simulink model "gm_Encoder_Zynq_V24"  (R2018a)
settings: Solver=ode3  StartTime=0.0  StopTime=SimulationsDauer  RelTol=1e-3  EnableMultiTasking=on
undefined symbols (not defined in the file or in its folder): DiscIntNeverNeededParam, f_ISR, IncPerTurn, n_max, OmegaPerOverSampl, OverSamplingFactor, OverSamplingFactorInverse, Periode, Phase_Delay_A, Phase_Delay_B, PolePair, QuadratureFactor, T_50MHz, T_mech, TestDrehzahl_rpm
libraries: simulink x2, dspswit3 x2, powerlib_meascontrol x2, simulink_extras x1, powerlib x1
(part 3 of 4)

== system gm_Encoder_Zynq_V24/IncreEncoder_V22/omega_by_measure_time ==
  note: Use new Speed after every positive A-Line Edge
  note: 1 for one cycle if edge recognized
  note: Detect each positive edge of the A-Line of the encoder
  note: Reset time measurement
  note: Count up in order to measure the time between to positive edges of the A-Line of the encoder
  Edge : Inport
  T : Inport  Port=2
  Add1 : Sum  OutDataTypeStr=Inherit: Same as first input
  Constant : Constant  Value=0  OutDataTypeStr=fixdt(0,32,26)  SampleTime=-1
  Constant1 : Constant  Value=0  OutDataTypeStr=fixdt(0,32,26)  SampleTime=-1
  Constant2 : Constant  Value=0  OutDataTypeStr=fixdt(0,32,26)  SampleTime=-1
  Constant3 : Constant  Value=0  OutDataTypeStr=int8  SampleTime=-1
  Detec_edge : Sum  Inputs=+-  AccumDataTypeStr=int8  OutDataTypeStr=int8
  ProtectOverflow_T_count : Switch  Threshold=50
  ProtectOverflow_rps : Switch  Threshold=50  OutDataTypeStr=fixdt(0,32,26)
  ProtectToUseOmegaIfThetaJump1 : RelationalOperator  Operator=>  OutDataTypeStr=boolean  RndMeth=Nearest
  Scope : Scope  NumInputPorts=3
  T_count : Delay  DelayLength=1
  T_count_switch : Switch  Criteria=u2 > Threshold
  count_old1 : Delay  DelayLength=1
  reset_old1 : Delay  DelayLength=1
  reset_old_switch1 : Switch  Criteria=u2 ~= 0
  speed_old : Delay  DelayLength=1
  speed_old_switch : Switch  Criteria=u2 ~= 0  OutDataTypeStr=fixdt(0,32,26)  RndMeth=Zero
  rps : Outport
  NewMeasurement : Outport  Port=2
  wires:
  Detec_edge/1 -> reset_old_switch1/2, count_old1/1  "1 for one cycle if edge recognized"
  reset_old1/1 -> Detec_edge/2, reset_old_switch1/3
  reset_old_switch1/1 -> reset_old1/1
  Edge/1 -> Detec_edge/1, reset_old_switch1/1
  ProtectToUseOmegaIfThetaJump1/1 -> T_count_switch/2, speed_old_switch/2, NewMeasurement/1, Scope/1
  Constant3/1 -> ProtectToUseOmegaIfThetaJump1/2
  count_old1/1 -> ProtectToUseOmegaIfThetaJump1/1
  T_count_switch/1 -> ProtectOverflow_T_count/2, ProtectOverflow_T_count/3, ProtectOverflow_rps/2
  Add1/1 -> T_count_switch/3, speed_old_switch/1, Scope/2
  T_count/1 -> Add1/2
  ProtectOverflow_T_count/1 -> T_count/1
  T/1 -> Add1/1
  speed_old/1 -> speed_old_switch/3
  speed_old_switch/1 -> speed_old/1, ProtectOverflow_rps/3
  Constant2/1 -> ProtectOverflow_rps/1
  ProtectOverflow_rps/1 -> rps/1, Scope/3
  Constant1/1 -> ProtectOverflow_T_count/1
  Constant/1 -> T_count_switch/1

== system gm_Encoder_Zynq_V24/IncreEncoder_V24/Check_Direction ==
  A : Inport  PortDimensions=1  SampleTime=2e-08
  B : Inport  Port=2  PortDimensions=1  SampleTime=2e-08
  Add : Sum  Inputs=+-  AccumDataTypeStr=fixdt(1, 4, 0)  OutDataTypeStr=fixdt(1, 4, 0)  SampleTime=2e-08
  Add1 : Sum  Inputs=+-  AccumDataTypeStr=fixdt(1, 4, 0)  OutDataTypeStr=fixdt(1, 4, 0)  SampleTime=2e-08
  Add2 : Sum  AccumDataTypeStr=fixdt(1, 4, 0)  OutDataTypeStr=fixdt(1, 4, 0)  SampleTime=2e-08
  Change : Sum  AccumDataTypeStr=fixdt(1, 4, 0)  OutDataTypeStr=fixdt(1, 4, 0)  SampleTime=2e-08
  Change1 : Delay  DelayLength=double(1)  InitialCondition=0  InputProcessing=Inherited  SampleTime=2e-08
  Save_Direction : Switch  Criteria=u2 ~= 0  Threshold=double(0)  OutDataTypeStr=fixdt(1, 4, 0)  SampleTime=2e-08
  T_count_switch : Switch  Threshold=double(1)  OutDataTypeStr=fixdt(1, 4, 0)  SampleTime=2e-08
  TrnLeft : Sum  Inputs=+-  AccumDataTypeStr=fixdt(1, 4, 0)  OutDataTypeStr=fixdt(1, 4, 0)  SampleTime=2e-08
  TrnRight : Sum  Inputs=+-  AccumDataTypeStr=fixdt(1, 4, 0)  OutDataTypeStr=fixdt(1, 4, 0)  SampleTime=2e-08
  TurnLeft : Constant  Value=fi(0,1,4,0,'hex','f')  OutDataTypeStr=fixdt(1, 4, 0)  SampleTime=-1
  TurnRight : Constant  Value=fi(0,1,4,0,'hex','1')  OutDataTypeStr=fixdt(1, 4, 0)  SampleTime=-1
  count_old : Delay  DelayLength=double(1)  InitialCondition=0  InputProcessing=Inherited  SampleTime=2e-08
  count_old1 : Delay  DelayLength=double(1)  InitialCondition=0  InputProcessing=Inherited  SampleTime=2e-08
  count_old2 : Delay  DelayLength=double(1)  InitialCondition=0  InputProcessing=Inherited  SampleTime=2e-08
  count_old_switch : Switch  Criteria=u2 ~= 0  Threshold=double(0)  OutDataTypeStr=boolean  SampleTime=2e-08
  count_old_switch1 : Switch  Criteria=u2 ~= 0  Threshold=double(0)  OutDataTypeStr=boolean  SampleTime=2e-08
  new_value : Delay  DelayLength=double(1)  InitialCondition=0  InputProcessing=Inherited  SampleTime=2e-08
  nothing : Constant  Value=fi(0,1,4,0,'hex','0')  OutDataTypeStr=fixdt(1, 4, 0)  SampleTime=-1
  nothing1 : Constant  Value=fi(0,1,4,0,'hex','0')  OutDataTypeStr=fixdt(1, 4, 0)  SampleTime=-1
  speed_old_switch : Switch  Threshold=double(1)  OutDataTypeStr=fixdt(1, 4, 0)  SampleTime=2e-08
  Dir : Outport
  wires:
  A/1 -> TrnLeft/2, Add/1, count_old_switch/1
  B/1 -> TrnRight/2, Add1/1, count_old_switch1/1
  Add/1 -> TrnRight/1, count_old_switch/2
  Add1/1 -> TrnLeft/1, count_old_switch1/2
  Add2/1 -> new_value/1
  Change/1 -> Change1/1
  Change1/1 -> Save_Direction/2
  T_count_switch/1 -> Change/1, Add2/1
  TrnLeft/1 -> speed_old_switch/2
  TrnRight/1 -> T_count_switch/2
  TurnLeft/1 -> speed_old_switch/1
  TurnRight/1 -> T_count_switch/1
  count_old2/1 -> Dir/1, Save_Direction/3
  new_value/1 -> Save_Direction/1
  nothing/1 -> speed_old_switch/3
  nothing1/1 -> T_count_switch/3
  speed_old_switch/1 -> Change/2, Add2/2
  count_old_switch/1 -> count_old/1
  count_old/1 -> count_old_switch/3, Add/2
  count_old_switch1/1 -> count_old1/1
  count_old1/1 -> count_old_switch1/3, Add1/2
  Save_Direction/1 -> count_old2/1

== system gm_Encoder_Zynq_V24/IncreEncoder_V24/Counter ==
  note: Reset
  note: 1 for one cycle if edge recognized
  Enable_ctr : Inport  PortDimensions=1  SampleTime=2e-08
  I_line : Inport  Port=2  PortDimensions=1  SampleTime=2e-08
  Detec_edge : Sum  Inputs=+-  AccumDataTypeStr=int8  OutDataTypeStr=int8  SampleTime=2e-08
  Reset_flag : Sum  Inputs=+-  AccumDataTypeStr=uint8  OutDataTypeStr=uint8  SampleTime=2e-08
  reset_old : Delay  DelayLength=double(1)  InitialCondition=0  InputProcessing=Inherited  SampleTime=2e-08
  reset_old1 : Delay  DelayLength=double(1)  InitialCondition=0  InputProcessing=Inherited  SampleTime=2e-08
  reset_old_switch : Switch  Criteria=u2 ~= 0  Threshold=double(0)  OutDataTypeStr=boolean  SampleTime=2e-08
  reset_old_switch1 : Switch  Criteria=u2 ~= 0  Threshold=double(0)  OutDataTypeStr=boolean  SampleTime=2e-08
  Edge : Outport
  Reset : Outport  Port=2
  wires:
  Enable_ctr/1 -> Detec_edge/1, reset_old_switch1/1
  I_line/1 -> Reset_flag/1, reset_old_switch/1
  Detec_edge/1 -> Edge/1, reset_old_switch1/2
  Reset_flag/1 -> Reset/1, reset_old_switch/2
  reset_old_switch1/1 -> reset_old1/1
  reset_old1/1 -> reset_old_switch1/3, Detec_edge/2
  reset_old_switch/1 -> reset_old/1
  reset_old/1 -> reset_old_switch/3, Reset_flag/2

== system gm_Encoder_Zynq_V24/IncreEncoder_V24/Counter_position ==
  note: Check if count is to small
  note: Check if count is to big 0-Increments
  note: Count
  Edge : Inport  PortDimensions=1  SampleTime=2e-08
  Reset : Inport  Port=2  PortDimensions=1  SampleTime=2e-08
  IncsPerTurn : Inport  Port=3  PortDimensions=1  SampleTime=2e-08
  Dir : Inport  Port=4  PortDimensions=1  SampleTime=2e-08
  Add1 : Sum  AccumDataTypeStr=int16  OutDataTypeStr=int16  SampleTime=2e-08
  Constant1 : Constant  Value=fi(0,1,16,0,'hex','0000')  OutDataTypeStr=int16  SampleTime=-1
  Constant2 : Constant  Value=fi(0,1,16,0,'hex','0001')  OutDataTypeStr=int16  SampleTime=-1
  Constant3 : Constant  Value=fi(0,1,16,0,'hex','0000')  OutDataTypeStr=int16  SampleTime=-1
  Constant5 : Constant  Value=fi(0,1,16,0,'hex','ffff')  OutDataTypeStr=int16  SampleTime=-1
  Relational Operator : RelationalOperator  Operator=>  OutDataTypeStr=boolean  SampleTime=2e-08  RndMeth=Nearest
  Relational Operator1 : RelationalOperator  Operator=<=  OutDataTypeStr=boolean  SampleTime=2e-08  RndMeth=Nearest
  Resett_switch1 : Switch  Criteria=u2 ~= 0  Threshold=double(0)  OutDataTypeStr=uint16  SampleTime=2e-08
  Resett_switch2 : Switch  Criteria=u2 ~= 0  Threshold=double(0)  OutDataTypeStr=int16  SampleTime=2e-08
  Resett_switch3 : Switch  Criteria=u2 ~= 0  Threshold=double(0)  OutDataTypeStr=int16  SampleTime=2e-08
  only_use_for_neg_speed : Switch  Threshold=double(1)  OutDataTypeStr=int16  SampleTime=2e-08
  reset_old{1..6} (6 alike) : Delay  DelayLength=double(1)  InitialCondition=0  InputProcessing=Inherited  SampleTime=2e-08
  speed_old_switch1 : Switch  Criteria=u2 ~= 0  Threshold=double(0)  OutDataTypeStr=int16  SampleTime=2e-08
  speed_old_switch2 : Switch  Threshold=double(1)  OutDataTypeStr=int16  SampleTime=2e-08
  count : Outport
  wires:
  Edge/1 -> speed_old_switch1/2
  Reset/1 -> Resett_switch2/2
  IncsPerTurn/1 -> reset_old5/1
  Dir/1 -> reset_old6/1
  Constant1/1 -> Relational Operator1/2, Resett_switch1/1, Resett_switch2/1, only_use_for_neg_speed/1
  Constant2/1 -> speed_old_switch2/1
  Constant3/1 -> speed_old_switch1/3
  Constant5/1 -> speed_old_switch2/3
  Resett_switch1/1 -> count/1, reset_old1/1, Relational Operator/1
  reset_old4/1 -> speed_old_switch1/1
  reset_old5/1 -> Relational Operator/2, Resett_switch3/1
  reset_old6/1 -> speed_old_switch2/2, only_use_for_neg_speed/2
  speed_old_switch1/1 -> Add1/1
  speed_old_switch2/1 -> reset_old4/1
  Resett_switch2/1 -> Resett_switch3/3
  Add1/1 -> Resett_switch2/3
  reset_old1/1 -> Add1/2
  Relational Operator1/1 -> reset_old2/1
  reset_old2/1 -> only_use_for_neg_speed/3
  only_use_for_neg_speed/1 -> Resett_switch3/2
  Resett_switch3/1 -> Resett_switch1/3, Relational Operator1/1
  Relational Operator/1 -> reset_old3/1
  reset_old3/1 -> Resett_switch1/2

== system gm_Encoder_Zynq_V24/IncreEncoder_V24/Counter_theta_ele ==
  note: Check if count is to small
  note: Count
  Edge : Inport  PortDimensions=1  SampleTime=2e-08
  Reset : Inport  Port=2  PortDimensions=1  SampleTime=2e-08
  IncsPerTurn : Inport  Port=3  PortDimensions=1  SampleTime=2e-08
  Dir : Inport  Port=4  PortDimensions=1  SampleTime=2e-08
  Add1 : Sum  AccumDataTypeStr=int16  OutDataTypeStr=int16  SampleTime=2e-08
  Constant1 : Constant  Value=fi(0,1,16,0,'hex','0000')  OutDataTypeStr=int16  SampleTime=-1
  Constant2 : Constant  Value=fi(0,1,16,0,'hex','0001')  OutDataTypeStr=int16  SampleTime=-1
  Constant3 : Constant  Value=fi(0,1,16,0,'hex','0000')  OutDataTypeStr=int16  SampleTime=-1
  Constant5 : Constant  Value=fi(0,1,16,0,'hex','ffff')  OutDataTypeStr=int16  SampleTime=-1
  Relational Operator : RelationalOperator  Operator=>  OutDataTypeStr=boolean  SampleTime=2e-08  RndMeth=Nearest
  Relational Operator1 : RelationalOperator  Operator=<=  OutDataTypeStr=boolean  SampleTime=2e-08  RndMeth=Nearest
  Reset_switch3 : Switch  Criteria=u2 ~= 0  Threshold=double(0)  OutDataTypeStr=int16  SampleTime=2e-08
  Resett_switch1 : Switch  Criteria=u2 ~= 0  Threshold=double(0)  OutDataTypeStr=int16  SampleTime=2e-08
  Resett_switch2 : Switch  Criteria=u2 ~= 0  Threshold=double(0)  OutDataTypeStr=int16  SampleTime=2e-08
  only_use_for_neg_speed : Switch  Threshold=double(1)  OutDataTypeStr=int16  SampleTime=2e-08
  reset_old{1..6} (6 alike) : Delay  DelayLength=double(1)  InitialCondition=0  InputProcessing=Inherited  SampleTime=2e-08
  speed_old_switch1 : Switch  Criteria=u2 ~= 0  Threshold=double(0)  OutDataTypeStr=int16  SampleTime=2e-08
  speed_old_switch2 : Switch  Threshold=double(1)  OutDataTypeStr=int16  SampleTime=2e-08
  count : Outport
  wires:
  Edge/1 -> speed_old_switch1/2
  Reset/1 -> Resett_switch2/2
  IncsPerTurn/1 -> reset_old1/1
  Dir/1 -> reset_old5/1
  Constant1/1 -> Relational Operator1/2, Resett_switch1/1, Resett_switch2/1, only_use_for_neg_speed/1
  Constant2/1 -> speed_old_switch2/1
  Constant3/1 -> speed_old_switch1/3
  Constant5/1 -> speed_old_switch2/3
  Resett_switch1/1 -> count/1, reset_old6/1, Relational Operator/1
  reset_old1/1 -> Relational Operator/2, Reset_switch3/1
  reset_old4/1 -> speed_old_switch1/1
  reset_old5/1 -> speed_old_switch2/2, only_use_for_neg_speed/2
  speed_old_switch1/1 -> Add1/1
  speed_old_switch2/1 -> reset_old4/1
  Resett_switch2/1 -> Reset_switch3/3
  Add1/1 -> Resett_switch2/3
  reset_old6/1 -> Add1/2
  Relational Operator1/1 -> reset_old2/1
  reset_old2/1 -> only_use_for_neg_speed/3
  only_use_for_neg_speed/1 -> Reset_switch3/2
  Reset_switch3/1 -> Resett_switch1/3, Relational Operator1/1
  Relational Operator/1 -> reset_old3/1
  reset_old3/1 -> Resett_switch1/2

== system gm_Encoder_Zynq_V24/IncreEncoder_V24/HDL Reciprocal ==
  In1 : Inport
  Delay1 : Delay  DelayLength=1  InputProcessing=Inherited
  Delay2 : Delay  DelayLength=3  InputProcessing=Inherited
  HDL Reciprocal : Reciprocal  SampleTime=2e-08
  Out1 : Outport
  wires:
  In1/1 -> Delay1/1
  Delay1/1 -> HDL Reciprocal/1
  HDL Reciprocal/1 -> Delay2/1
  Delay2/1 -> Out1/1

== system gm_Encoder_Zynq_V24/IncreEncoder_V24/omega_by_count_lines ==
  note: Count
  note: Check if count is to big in order to safe for value overflow
  note: Set new counter value
  Edge : Inport  PortDimensions=1  SampleTime=2e-08
  Reset : Inport  Port=2  PortDimensions=1  SampleTime=2e-08
  IncsPerTurn : Inport  Port=3  PortDimensions=1  SampleTime=2e-08
  Add1 : Sum  AccumDataTypeStr=int16  OutDataTypeStr=int16  SampleTime=2e-08
  Constant1 : Constant  Value=fi(0,1,16,0,'hex','0000')  OutDataTypeStr=int16  SampleTime=-1
  Constant2 : Constant  Value=fi(0,1,16,0,'hex','0001')  OutDataTypeStr=int16  SampleTime=-1
  Constant3 : Constant  Value=fi(0,1,16,0,'hex','0000')  OutDataTypeStr=int16  SampleTime=-1
  Constant4 : Constant  Value=fi(0,1,16,0,'hex','000a')  OutDataTypeStr=int16  SampleTime=-1
  Relational Operator : RelationalOperator  Operator=>  OutDataTypeStr=boolean  SampleTime=2e-08  RndMeth=Nearest
  Reset_when_overflow : Sum  AccumDataTypeStr=fixdt(1, 18, 0)  OutDataTypeStr=int16  SampleTime=2e-08
  Resett_switch1 : Switch  Criteria=u2 ~= 0  Threshold=double(0)  OutDataTypeStr=int16  SampleTime=2e-08
  Resett_switch2 : Switch  Criteria=u2 ~= 0  Threshold=double(0)  OutDataTypeStr=int16  SampleTime=2e-08
  reset_old{1,3..5} (4 alike) : Delay  DelayLength=double(1)  InitialCondition=0  InputProcessing=Inherited  SampleTime=2e-08
  reset_old_switch1 : Switch  Criteria=u2 ~= 0  Threshold=double(0)  OutDataTypeStr=int16  SampleTime=2e-08
  speed_old_switch1 : Switch  Criteria=u2 ~= 0  Threshold=double(0)  OutDataTypeStr=int16  SampleTime=2e-08
  count : Outport
  wires:
  Edge/1 -> speed_old_switch1/2
  Reset/1 -> Resett_switch2/2, reset_old_switch1/2
  IncsPerTurn/1 -> Reset_when_overflow/2
  Constant1/1 -> Resett_switch1/1, Resett_switch2/1
  Constant2/1 -> reset_old4/1
  Constant3/1 -> speed_old_switch1/3
  Constant4/1 -> Reset_when_overflow/1
  Reset_when_overflow/1 -> reset_old5/1
  reset_old3/1 -> Add1/2, Relational Operator/1, reset_old_switch1/1
  reset_old4/1 -> speed_old_switch1/1
  reset_old5/1 -> Relational Operator/2
  reset_old_switch1/1 -> count/1, reset_old1/1
  speed_old_switch1/1 -> Add1/1
  Resett_switch2/1 -> Resett_switch1/3
  Add1/1 -> Resett_switch2/3
  Relational Operator/1 -> Resett_switch1/2
  Resett_switch1/1 -> reset_old3/1
  reset_old1/1 -> reset_old_switch1/3

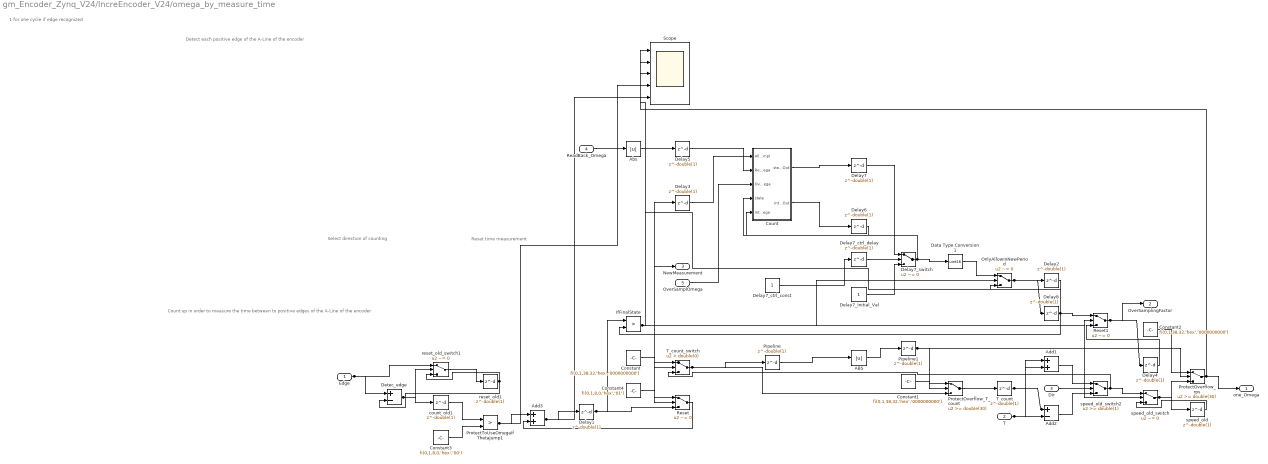
== system gm_Encoder_Zynq_V24/IncreEncoder_V24/omega_by_measure_time ==
  note: Select direction of counting
  note: 1 for one cycle if edge recognized
  note: Detect each positive edge of the A-Line of the encoder
  note: Reset time measurement
  note: Count up in order to measure the time between to positive edges of the A-Line of the encoder
  Edge : Inport  PortDimensions=1  SampleTime=2e-08
  T : Inport  Port=2  PortDimensions=1  SampleTime=2e-08
  Dir : Inport  Port=3  PortDimensions=1  SampleTime=2e-08
  ReadBack_Omega : Inport  Port=4  PortDimensions=1  SampleTime=2e-08
  OverSamplOmega : Inport  Port=5  PortDimensions=1  SampleTime=2e-08
  ABS : Abs  SampleTime=2e-08  OutDataTypeStr=fixdt(1, 38, 32)
  Abs : Abs  SampleTime=2e-08  OutDataTypeStr=fixdt(1, 24, 11)
  Add1 : Sum  AccumDataTypeStr=fixdt(1, 38, 32)  OutDataTypeStr=fixdt(1, 38, 32)  SampleTime=2e-08
  Add2 : Sum  Inputs=+-  AccumDataTypeStr=fixdt(1, 38, 32)  OutDataTypeStr=fixdt(1, 38, 32)  SampleTime=2e-08
  Add3 : Sum  AccumDataTypeStr=int16  OutDataTypeStr=int16  SampleTime=2e-08
  Constant : Constant  Value=fi(0,1,38,32,'hex','0000000000')  OutDataTypeStr=fixdt(1, 38, 32)  SampleTime=-1
  Constant1 : Constant  Value=fi(0,1,38,32,'hex','0000000000')  OutDataTypeStr=fixdt(1, 38, 32)  SampleTime=-1
  Constant2 : Constant  Value=fi(0,1,38,32,'hex','0000000000')  OutDataTypeStr=fixdt(1, 38, 32)  SampleTime=-1
  Constant3 : Constant  Value=fi(0,1,8,0,'hex','00')  OutDataTypeStr=int8  SampleTime=-1
  Constant4 : Constant  Value=fi(0,1,8,0,'hex','01')  OutDataTypeStr=int8  SampleTime=-1
  Count : Subsystem
  Data Type Conversion1 : DataTypeConversion  OutDataTypeStr=uint16  SampleTime=2e-08
  Delay{1..8} (8 alike) : Delay  DelayLength=double(1)  InitialCondition=0  InputProcessing=Inherited  SampleTime=2e-08
  Delay7_Initial_Val : Constant  OutDataTypeStr=uint16  SampleTime=-1
  Delay7_ctrl_const : Constant  OutDataTypeStr=boolean  SampleTime=2e-08
  Delay7_ctrl_delay : Delay  DelayLength=double(1)  InitialCondition=0  InputProcessing=Inherited  SampleTime=2e-08
  Delay7_switch : Switch  Criteria=u2 ~= 0  Threshold=double(0)  OutDataTypeStr=uint16  SampleTime=2e-08
  Detec_edge : Sum  Inputs=+-  AccumDataTypeStr=int8  OutDataTypeStr=int8  SampleTime=2e-08
  IfFinalState : RelationalOperator  Operator=>  OutDataTypeStr=boolean  SampleTime=2e-08  RndMeth=Nearest
  OnlyAllowInNewPeriod : Switch  Criteria=u2 ~= 0  Threshold=double(0)  OutDataTypeStr=uint16  SampleTime=2e-08
  Pipeline : Delay  DelayLength=double(1)  InitialCondition=0  InputProcessing=Inherited  SampleTime=2e-08
  Pipeline1 : Delay  DelayLength=double(1)  InitialCondition=0  InputProcessing=Inherited  SampleTime=2e-08
  ProtectOverflow_T_count : Switch  Threshold=double(30)  OutDataTypeStr=fixdt(1, 38, 32)  SampleTime=2e-08
  ProtectOverflow_rps : Switch  Threshold=double(30)  OutDataTypeStr=fixdt(1, 38, 32)  SampleTime=2e-08
  ProtectToUseOmegaIfThetaJump1 : RelationalOperator  Operator=>  SampleTime=2e-08  RndMeth=Nearest
  Reset : Switch  Criteria=u2 ~= 0  Threshold=double(0)  OutDataTypeStr=fixdt(1, 24, 11)  SampleTime=2e-08
  Reset1 : Switch  Criteria=u2 ~= 0  Threshold=double(0)  OutDataTypeStr=uint16  SampleTime=2e-08
  Scope : Scope  NumInputPorts=5
  T_count : Delay  DelayLength=double(1)  InitialCondition=0  InputProcessing=Inherited  SampleTime=2e-08
  T_count_switch : Switch  Criteria=u2 > Threshold  Threshold=double(0)  OutDataTypeStr=fixdt(1, 38, 32)  SampleTime=2e-08
  count_old1 : Delay  DelayLength=double(1)  InitialCondition=0  InputProcessing=Inherited  SampleTime=2e-08
  reset_old1 : Delay  DelayLength=double(1)  InitialCondition=0  InputProcessing=Inherited  SampleTime=2e-08
  reset_old_switch1 : Switch  Criteria=u2 ~= 0  Threshold=double(0)  OutDataTypeStr=boolean  SampleTime=2e-08
  speed_old : Delay  DelayLength=double(1)  InitialCondition=0  InputProcessing=Inherited  SampleTime=2e-08
  speed_old_switch : Switch  Criteria=u2 ~= 0  Threshold=double(0)  OutDataTypeStr=fixdt(1, 38, 32)  SampleTime=2e-08
  speed_old_switch2 : Switch  Threshold=double(1)  OutDataTypeStr=fixdt(1, 38, 32)  SampleTime=2e-08
  one_Omega : Outport
  OverSamplingFactor : Outport  Port=2
  NewMeasurement : Outport  Port=3
  wires:
  Edge/1 -> reset_old_switch1/1, Detec_edge/1
  T/1 -> Add2/2, Add1/2
  Dir/1 -> speed_old_switch2/2
  ReadBack_Omega/1 -> Abs/1
  OverSamplOmega/1 -> Count/3(OverSamplOmega)
  ABS/1 -> Pipeline1/1
  Abs/1 -> Delay5/1
  Add1/1 -> speed_old_switch2/1
  Add2/1 -> speed_old_switch2/3
  Add3/1 -> Scope/5, Delay1/1
  Constant/1 -> T_count_switch/1
  Constant1/1 -> ProtectOverflow_T_count/1
  Constant2/1 -> ProtectOverflow_rps/1
  Constant3/1 -> ProtectToUseOmegaIfThetaJump1/2
  Constant4/1 -> Reset/1
  Count/1(state_Out) -> Delay7/1
  Count/2(InternalOmega_Out) -> Delay6/1
  Data Type Conversion1/1 -> OnlyAllowInNewPeriod/1
  Delay1/1 -> Reset/3, IfFinalState/1
  Delay2/1 -> OnlyAllowInNewPeriod/3
  Delay3/1 -> Count/1(AllowCheckOverSampl)
  Delay4/1 -> Reset1/3
  Delay5/1 -> Count/2(ReadBack_Omega)
  Delay6/1 -> Count/5(InternalOmega)
  Delay7_switch/1 -> Data Type Conversion1/1, Count/4(state)
  Delay8/1 -> Reset1/1, IfFinalState/2, Scope/2
  Detec_edge/1 -> reset_old_switch1/2, count_old1/1
  IfFinalState/1 -> speed_old_switch/2, T_count_switch/2, Reset1/2, Reset/2, OnlyAllowInNewPeriod/2, Scope/1, Delay3/1, NewMeasurement/1
  OnlyAllowInNewPeriod/1 -> Delay8/1, Delay2/1
  Pipeline/1 -> ABS/1
  Pipeline1/1 -> ProtectOverflow_rps/2, ProtectOverflow_T_count/2
  ProtectOverflow_T_count/1 -> T_count/1
  ProtectOverflow_rps/1 -> Scope/3, one_Omega/1
  ProtectToUseOmegaIfThetaJump1/1 -> Add3/1, Scope/4
  Reset/1 -> Add3/2
  Reset1/1 -> Delay4/1, OverSamplingFactor/1
  T_count/1 -> Add2/1, Add1/1
  T_count_switch/1 -> ProtectOverflow_T_count/3, Pipeline/1
  count_old1/1 -> ProtectToUseOmegaIfThetaJump1/1
  reset_old1/1 -> reset_old_switch1/3, Detec_edge/2
  reset_old_switch1/1 -> reset_old1/1
  speed_old/1 -> speed_old_switch/3
  speed_old_switch/1 -> ProtectOverflow_rps/3, speed_old/1
  speed_old_switch2/1 -> speed_old_switch/1, T_count_switch/3
  Delay7/1 -> Delay7_switch/1
  Delay7_Initial_Val/1 -> Delay7_switch/3
  Delay7_ctrl_const/1 -> Delay7_ctrl_delay/1
  Delay7_ctrl_delay/1 -> Delay7_switch/2

== system gm_Encoder_Zynq_V24/IncreEncoder_V24_Gut/Average ==
  note: Maximum of the OverSampling is 6
  "OmegaIn " : Inport
  NewMeasurement : Inport  Port=2
  SamplingFactorInv : Inport  Port=3
  SamplingFactor : Inport  Port=4
  Add : Sum  Inputs=++++++  AccumDataTypeStr=fixdt(1,26,11)  OutDataTypeStr=fixdt(1,25,11)
  Ask1 : Switch  Threshold=fi(2,0,4,0)  OutDataTypeStr=fixdt(1,24,11)
  Ask2 : Switch  Threshold=fi(3,0,4,0)  OutDataTypeStr=fixdt(1,24,11)
  Ask3 : Switch  Threshold=fi(4,0,4,0)  OutDataTypeStr=fixdt(1,24,11)
  Ask4 : Switch  Threshold=fi(5,0,4,0)  OutDataTypeStr=fixdt(1,24,11)
  Ask5 : Switch  Threshold=fi(6,0,4,0)  OutDataTypeStr=fixdt(1,24,11)
  Constant1 : Constant  Value=0  OutDataTypeStr=fixdt(1,24,11)  SampleTime=-1
  NewSpeed{,1..4} (5 alike) : Switch  Criteria=u2 ~= 0  Threshold=0.5  OutDataTypeStr=fixdt(1,24,11)
  Product : Product  OutDataTypeStr=fixdt(1,24,11)
  hold{,1..4} (5 alike) : Delay  DelayLength=1
  OmegaOut : Outport
  wires:
  SamplingFactor/1 -> Ask5/2, Ask4/2, Ask3/2, Ask2/2, Ask1/2
  Ask5/1 -> Add/6
  Ask4/1 -> Add/5
  Ask3/1 -> Add/4
  Ask2/1 -> Add/3
  Ask1/1 -> Add/2
  Constant1/1 -> Ask1/3, Ask2/3, Ask3/3, Ask4/3, Ask5/3
  hold4/1 -> NewSpeed4/3
  NewSpeed4/1 -> Ask5/1, hold4/1
  hold3/1 -> NewSpeed3/3, NewSpeed4/1
  NewSpeed3/1 -> Ask4/1, hold3/1
  NewMeasurement/1 -> NewSpeed1/2, NewSpeed2/2, NewSpeed3/2, NewSpeed4/2, NewSpeed/2
  NewSpeed2/1 -> Ask3/1, hold2/1
  hold2/1 -> NewSpeed2/3, NewSpeed3/1
  hold1/1 -> NewSpeed1/3, NewSpeed2/1
  NewSpeed1/1 -> Ask2/1, hold1/1
  NewSpeed/1 -> Ask1/1, hold/1
  hold/1 -> NewSpeed/3, NewSpeed1/1
  Add/1 -> Product/1
  SamplingFactorInv/1 -> Product/2
  "OmegaIn "/1 -> NewSpeed/1, Add/1
  Product/1 -> OmegaOut/1

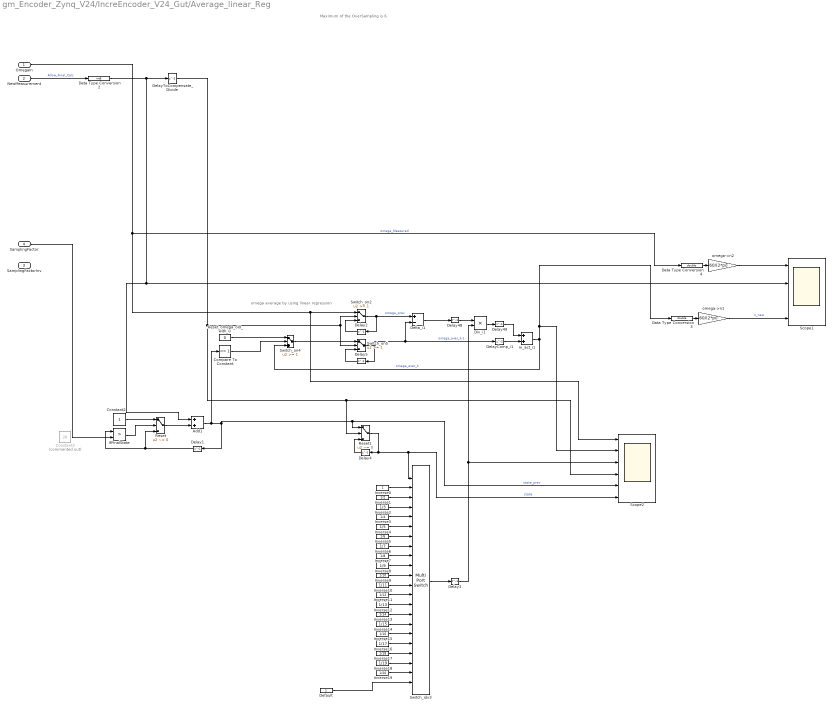
== system gm_Encoder_Zynq_V24/IncreEncoder_V24_Gut/Average_linear_Reg ==
  note: omega average by using linear regression
  note: Maximum of the OverSampling is 6
  "OmegaIn " : Inport
  NewMeasurement : Inport  Port=2
  SamplingFactorInv : Inport  Port=3
  SamplingFactor : Inport  Port=4
  Add1 : Sum  OutDataTypeStr=Inherit: Same as accumulator
  Compare To Constant : simulink/Logic and Bit Operations/Compare To Constant  relop===  const=1  OutDataTypeStr=boolean
  Constant2 : Constant  OutDataTypeStr=int8  SampleTime=T_50MHz
  Constant3 : Constant  Commented=on  Value=20  OutDataTypeStr=uint16  SampleTime=T_50MHz
  Data Type Conversion2 : DataTypeConversion  OutDataTypeStr=int8
  Data Type Conversion3 : DataTypeConversion  OutDataTypeStr=double
  Data Type Conversion4 : DataTypeConversion  OutDataTypeStr=double
  Default : Constant  OutDataTypeStr=fixdt(0,18,18)  SampleTime=-1
  Delay{1..5,48..49} (7 alike) : Delay  DelayLength=1  InitialCondition=0
  DelayComp_i1 : Delay  InitialCondition=0
  DelayToCompensate_Divide : Delay
  Delta_i1 : Sum  Inputs=+-  AccumDataTypeStr=fixdt(1,32,18)  OutDataTypeStr=fixdt(1,24,11)
  Div_i1 : Product  Inputs=**  RndMeth=Simplest  SaturateOnIntegerOverflow=on  OutDataTypeStr=Inherit: Same as first input
  IfFinalState : RelationalOperator  Operator=>  OutDataTypeStr=boolean  RndMeth=Nearest
  Inverse0 : Constant  OutDataTypeStr=fixdt(0,18,18)  SampleTime=-1
  Inverse1 : Constant  Value=1/2  OutDataTypeStr=fixdt(0,18,18)  SampleTime=-1
  Inverse10 : Constant  Value=1/11  OutDataTypeStr=fixdt(0,18,18)  SampleTime=-1
  Inverse11 : Constant  Value=1/12  OutDataTypeStr=fixdt(0,18,18)  SampleTime=-1
  Inverse12 : Constant  Value=1/13  OutDataTypeStr=fixdt(0,18,18)  SampleTime=-1
  Inverse13 : Constant  Value=1/14  OutDataTypeStr=fixdt(0,18,18)  SampleTime=-1
  Inverse14 : Constant  Value=1/15  OutDataTypeStr=fixdt(0,18,18)  SampleTime=-1
  Inverse15 : Constant  Value=1/16  OutDataTypeStr=fixdt(0,18,18)  SampleTime=-1
  Inverse16 : Constant  Value=1/17  OutDataTypeStr=fixdt(0,18,18)  SampleTime=-1
  Inverse17 : Constant  Value=1/18  OutDataTypeStr=fixdt(0,18,18)  SampleTime=-1
  Inverse18 : Constant  Value=1/19  OutDataTypeStr=fixdt(0,18,18)  SampleTime=-1
  Inverse19 : Constant  Value=1/20  OutDataTypeStr=fixdt(0,18,18)  SampleTime=-1
  Inverse2 : Constant  Value=1/3  OutDataTypeStr=fixdt(0,18,18)  SampleTime=-1
  Inverse3 : Constant  Value=1/4  OutDataTypeStr=fixdt(0,18,18)  SampleTime=-1
  Inverse4 : Constant  Value=1/5  OutDataTypeStr=fixdt(0,18,18)  SampleTime=-1
  Inverse5 : Constant  Value=1/6  OutDataTypeStr=fixdt(0,18,18)  SampleTime=-1
  Inverse6 : Constant  Value=1/7  OutDataTypeStr=fixdt(0,18,18)  SampleTime=-1
  Inverse7 : Constant  Value=1/8  OutDataTypeStr=fixdt(0,18,18)  SampleTime=-1
  Inverse8 : Constant  Value=1/9  OutDataTypeStr=fixdt(0,18,18)  SampleTime=-1
  Inverse9 : Constant  Value=1/10  OutDataTypeStr=fixdt(0,18,18)  SampleTime=-1
  Reset : Switch  Criteria=u2 ~= 0  Threshold=0.5  OutDataTypeStr=fixdt(1,24,11)
  Reset1 : Switch  Criteria=u2 ~= 0  Threshold=0.5  OutDataTypeStr=fixdt(1,24,11)
  Reset_omega_old_with_0 : Constant  Value=0  OutDataTypeStr=fixdt(1,24,11)  SampleTime=-1
  Scope1 : Scope  NumInputPorts=4
  Scope2 : Scope  NumInputPorts=6
  Switch_idx3 : MultiPortSwitch  Inputs=20  DataPortForDefault=Additional data port  DiagnosticForDefault=None  OutDataTypeStr=fixdt(0,18,18)  RndMeth=Simplest
  Switch_on2 : Switch  Threshold=1  OutDataTypeStr=fixdt(1,24,11)  RndMeth=Simplest
  Switch_on4 : Switch  Threshold=1  OutDataTypeStr=Inherit: Inherit via back propagation  RndMeth=Simplest
  Switch_on5 : Switch  Threshold=1  OutDataTypeStr=Inherit: Inherit via back propagation  RndMeth=Simplest
  m_act_i1 : Sum  OutDataTypeStr=Inherit: Same as accumulator  RndMeth=Simplest
  omega->n1 : Gain  Gain=60/(2*pi)  OutDataTypeStr=double
  omega->n2 : Gain  Gain=60/(2*pi)  OutDataTypeStr=double
  wires:
  SamplingFactor/1 -> IfFinalState/2
  Compare To Constant/1 -> Switch_on4/2
  omega->n2/1 -> Scope1/1
  Data Type Conversion4/1 -> omega->n2/1
  DelayToCompensate_Divide/1 -> Switch_on2/2, Switch_on5/2, Reset1/2, Scope2/4
  Delay4/1 -> Reset1/3
  Reset1/1 -> Delay4/1, Switch_idx3/1, Scope2/6  "state"
  Delay3/1 -> Scope2/3, Div_i1/2
  Switch_idx3/1 -> Delay3/1
  Switch_on4/1 -> Switch_on5/1
  Reset_omega_old_with_0/1 -> Switch_on4/1
  omega->n1/1 -> Scope1/4  "n_new"
  Data Type Conversion3/1 -> omega->n1/1
  Delay1/1 -> IfFinalState/1, Reset/3
  Data Type Conversion2/1 -> DelayToCompensate_Divide/1, Scope1/2, Add1/1
  Constant2/1 -> Reset/1
  Reset/1 -> Add1/2
  IfFinalState/1 -> Reset/2
  Add1/1 -> Compare To Constant/1, Delay1/1, Reset1/1, Scope2/5  "state_prev"
  Inverse1/1 -> Switch_idx3/3
  Default/1 -> Switch_idx3/22
  Inverse13/1 -> Switch_idx3/15
  Inverse12/1 -> Switch_idx3/14
  Inverse9/1 -> Switch_idx3/11
  Inverse3/1 -> Switch_idx3/5
  Inverse19/1 -> Switch_idx3/21
  Inverse8/1 -> Switch_idx3/10
  Inverse17/1 -> Switch_idx3/19
  Inverse2/1 -> Switch_idx3/4
  Inverse5/1 -> Switch_idx3/7
  Inverse6/1 -> Switch_idx3/8
  Inverse4/1 -> Switch_idx3/6
  Inverse15/1 -> Switch_idx3/17
  Inverse0/1 -> Switch_idx3/2
  Inverse18/1 -> Switch_idx3/20
  Inverse16/1 -> Switch_idx3/18
  Inverse7/1 -> Switch_idx3/9
  Inverse10/1 -> Switch_idx3/12
  Inverse11/1 -> Switch_idx3/13
  Inverse14/1 -> Switch_idx3/16
  Delay2/1 -> Switch_on2/3
  Switch_on2/1 -> Delta_i1/1, Delay2/1  "omega_prev"
  Div_i1/1 -> Delay49/1
  Delay48/1 -> Div_i1/1
  Delta_i1/1 -> Delay48/1
  Delay49/1 -> m_act_i1/1
  Switch_on5/1 -> Delay5/1, Delta_i1/2, DelayComp_i1/1  "omega_aver_k-1"
  m_act_i1/1 -> Data Type Conversion3/1, Scope2/2, Switch_on4/3  "omega_aver_k"
  "OmegaIn "/1 -> Switch_on2/1, Scope2/1, Data Type Conversion4/1  "omega_Measured"
  DelayComp_i1/1 -> m_act_i1/2
  NewMeasurement/1 -> Data Type Conversion2/1  "Allow_Final_Calc"
  Delay5/1 -> Switch_on5/3

== system gm_Encoder_Zynq_V24/IncreEncoder_V24_Gut/Check_Direction ==
  A : Inport
  B : Inport  Port=2
  Add : Sum  Inputs=+-  AccumDataTypeStr=fixdt(1,4,0)  OutDataTypeStr=fixdt(1,4,0)
  Add1 : Sum  Inputs=+-  AccumDataTypeStr=fixdt(1,4,0)  OutDataTypeStr=fixdt(1,4,0)
  Add2 : Sum  AccumDataTypeStr=fixdt(1,4,0)  OutDataTypeStr=fixdt(1,4,0)
  Change : Sum  AccumDataTypeStr=fixdt(1,4,0)  OutDataTypeStr=fixdt(1,4,0)
  Change1 : Delay  DelayLength=1
  Save_Direction : Switch  Criteria=u2 ~= 0  Threshold=0.1  OutDataTypeStr=fixdt(1,4,0)
  T_count_switch : Switch  Threshold=1  OutDataTypeStr=Inherit: Inherit via back propagation
  TrnLeft : Sum  Inputs=+-  AccumDataTypeStr=fixdt(1,4,0)  OutDataTypeStr=fixdt(1,4,0)
  TrnRight : Sum  Inputs=+-  AccumDataTypeStr=fixdt(1,4,0)  OutDataTypeStr=fixdt(1,4,0)
  TurnLeft : Constant  Value=-1  OutDataTypeStr=fixdt(1,4,0)  SampleTime=-1
  TurnRight : Constant  OutDataTypeStr=fixdt(1,4,0)  SampleTime=-1
  count_old : Delay  DelayLength=1
  count_old1 : Delay  DelayLength=1
  count_old2 : Delay  DelayLength=1
  count_old_switch : Switch  Criteria=u2 ~= 0  OutDataTypeStr=Inherit: Inherit via back propagation
  count_old_switch1 : Switch  Criteria=u2 ~= 0  OutDataTypeStr=Inherit: Inherit via back propagation
  new_value : Delay  DelayLength=1
  nothing : Constant  Value=0  OutDataTypeStr=fixdt(1,4,0)  SampleTime=-1
  nothing1 : Constant  Value=0  OutDataTypeStr=fixdt(1,4,0)  SampleTime=-1
  speed_old_switch : Switch  Threshold=1  OutDataTypeStr=Inherit: Inherit via back propagation
  Dir : Outport
  wires:
  count_old2/1 -> Dir/1, Save_Direction/3  "Dir"
  Change1/1 -> Save_Direction/2  "Change"
  Change/1 -> Change1/1
  Add2/1 -> new_value/1
  speed_old_switch/1 -> Add2/2, Change/2
  nothing1/1 -> T_count_switch/3
  nothing/1 -> speed_old_switch/3
  TurnLeft/1 -> speed_old_switch/1
  TrnLeft/1 -> speed_old_switch/2  "TrnLeft"
  new_value/1 -> Save_Direction/1
  TrnRight/1 -> T_count_switch/2  "Trn_Right"
  Add1/1 -> count_old_switch1/2, TrnLeft/1  "Edge_B"
  count_old1/1 -> Add1/2, count_old_switch1/3
  count_old_switch1/1 -> count_old1/1
  B/1 -> count_old_switch1/1, Add1/1, TrnRight/2
  Save_Direction/1 -> count_old2/1
  T_count_switch/1 -> Add2/1, Change/1
  Add/1 -> count_old_switch/2, TrnRight/1  "Edge_A"
  TurnRight/1 -> T_count_switch/1
  count_old/1 -> Add/2, count_old_switch/3
  count_old_switch/1 -> count_old/1
  A/1 -> count_old_switch/1, Add/1, TrnLeft/2

== system gm_Encoder_Zynq_V24/IncreEncoder_V24_Gut/Counter ==
  note: Reset
  note: 1 for one cycle if edge recognized
  Enable_ctr : Inport
  I_line : Inport  Port=2
  Detec_edge : Sum  Inputs=+-  AccumDataTypeStr=int8  OutDataTypeStr=int8
  Reset_flag : Sum  Inputs=+-  AccumDataTypeStr=uint8  OutDataTypeStr=uint8
  reset_old : Delay  DelayLength=1
  reset_old1 : Delay  DelayLength=1
  reset_old_switch : Switch  Criteria=u2 ~= 0
  reset_old_switch1 : Switch  Criteria=u2 ~= 0
  Edge : Outport
  Reset : Outport  Port=2
  wires:
  Detec_edge/1 -> Edge/1, reset_old_switch1/2  "1 for one cycle if edge recognized"
  reset_old1/1 -> Detec_edge/2, reset_old_switch1/3
  reset_old_switch1/1 -> reset_old1/1
  Enable_ctr/1 -> reset_old_switch1/1, Detec_edge/1
  Reset_flag/1 -> reset_old_switch/2, Reset/1
  reset_old/1 -> Reset_flag/2, reset_old_switch/3
  reset_old_switch/1 -> reset_old/1
  I_line/1 -> reset_old_switch/1, Reset_flag/1

== system gm_Encoder_Zynq_V24/IncreEncoder_V24_Gut/Counter_position ==
  note: Check if count is to small
  note: Check if count is to big 0-Increments
  note: Count
  Edge : Inport
  Reset : Inport  Port=2
  IncsPerTurn : Inport  Port=3
  Dir : Inport  Port=4
  Add1 : Sum  AccumDataTypeStr=int16  OutDataTypeStr=int16
  Constant1 : Constant  Value=0  OutDataTypeStr=int16  SampleTime=-1
  Constant2 : Constant  OutDataTypeStr=int16  SampleTime=-1
  Constant3 : Constant  Value=0  OutDataTypeStr=int16  SampleTime=-1
  Constant5 : Constant  Value=-1  OutDataTypeStr=int16  SampleTime=-1
  Relational Operator : RelationalOperator  Operator=>  OutDataTypeStr=boolean  RndMeth=Nearest
  Relational Operator1 : RelationalOperator  Operator=<=  OutDataTypeStr=boolean  RndMeth=Nearest
  Resett_switch1 : Switch  Criteria=u2 ~= 0  OutDataTypeStr=uint16
  Resett_switch2 : Switch  Criteria=u2 ~= 0  OutDataTypeStr=int16
  Resett_switch3 : Switch  Criteria=u2 ~= 0  OutDataTypeStr=int16
  only_use_for_neg_speed : Switch  Threshold=1
  reset_old{1..6} (6 alike) : Delay  DelayLength=1
  speed_old_switch1 : Switch  Criteria=u2 ~= 0
  speed_old_switch2 : Switch  Threshold=1
  count : Outport
  wires:
  reset_old1/1 -> Add1/2
  reset_old5/1 -> Resett_switch3/1, Relational Operator/2
  reset_old2/1 -> only_use_for_neg_speed/3
  reset_old3/1 -> Resett_switch1/2
  Resett_switch1/1 -> count/1, reset_old1/1, Relational Operator/1
  reset_old6/1 -> speed_old_switch2/2, only_use_for_neg_speed/2
  IncsPerTurn/1 -> reset_old5/1
  reset_old4/1 -> speed_old_switch1/1
  only_use_for_neg_speed/1 -> Resett_switch3/2
  Relational Operator1/1 -> reset_old2/1
  Resett_switch3/1 -> Resett_switch1/3, Relational Operator1/1
  Resett_switch2/1 -> Resett_switch3/3
  Constant1/1 -> Resett_switch2/1, Relational Operator1/2, only_use_for_neg_speed/1, Resett_switch1/1
  Relational Operator/1 -> reset_old3/1
  speed_old_switch2/1 -> reset_old4/1
  Constant5/1 -> speed_old_switch2/3
  Dir/1 -> reset_old6/1
  Constant2/1 -> speed_old_switch2/1
  Constant3/1 -> speed_old_switch1/3
  speed_old_switch1/1 -> Add1/1
  Add1/1 -> Resett_switch2/3
  Edge/1 -> speed_old_switch1/2  "1 for one cycle if edge recognized"
  Reset/1 -> Resett_switch2/2

== system gm_Encoder_Zynq_V24/IncreEncoder_V24_Gut/Counter_theta_ele ==
  note: Check if count is to small
  note: Check if count is to big
      | -Count from 0-Increments
      | - e.g. for 5000 increments, 4 pole pairs and A/B-Line (quadrature),
      | we count from 0-(5000*4/4) = 0-5000
      | - In that case, we must reset to 0, as soon as we have a value,
      | which is 1 bigger than increments (e.g. 5001 = 0).
  note: Count
  note: This Reset (I-Line) synchronize only
      | theta with position.
      | Since I-Line comes only once per
      | mechanical turn. Normaly the "IncsPerTurn"
      | do the Reset.
  Edge : Inport
  Reset : Inport  Port=2
  IncsPerTurn : Inport  Port=3
  Dir : Inport  Port=4
  Add1 : Sum  AccumDataTypeStr=int16  OutDataTypeStr=int16
  Constant1 : Constant  Value=0  OutDataTypeStr=int16  SampleTime=-1
  Constant2 : Constant  OutDataTypeStr=int16  SampleTime=-1
  Constant3 : Constant  Value=0  OutDataTypeStr=int16  SampleTime=-1
  Constant5 : Constant  Value=-1  OutDataTypeStr=int16  SampleTime=-1
  Relational Operator : RelationalOperator  Operator=>  OutDataTypeStr=boolean  RndMeth=Nearest
  Relational Operator1 : RelationalOperator  Operator=<=  OutDataTypeStr=boolean  RndMeth=Nearest
  Reset_switch3 : Switch  Criteria=u2 ~= 0  OutDataTypeStr=int16
  Resett_switch1 : Switch  Criteria=u2 ~= 0  OutDataTypeStr=int16
  Resett_switch2 : Switch  Criteria=u2 ~= 0  OutDataTypeStr=int16
  only_use_for_neg_speed : Switch  Threshold=1
  reset_old{1..6} (6 alike) : Delay  DelayLength=1
  speed_old_switch1 : Switch  Criteria=u2 ~= 0
  speed_old_switch2 : Switch  Threshold=1
  count : Outport
  wires:
  reset_old6/1 -> Add1/2
  reset_old1/1 -> Reset_switch3/1, Relational Operator/2
  reset_old2/1 -> only_use_for_neg_speed/3
  reset_old3/1 -> Resett_switch1/2
  reset_old5/1 -> only_use_for_neg_speed/2, speed_old_switch2/2
  reset_old4/1 -> speed_old_switch1/1
  only_use_for_neg_speed/1 -> Reset_switch3/2
  Relational Operator1/1 -> reset_old2/1
  Reset_switch3/1 -> Resett_switch1/3, Relational Operator1/1
  Resett_switch2/1 -> Reset_switch3/3
  Constant1/1 -> Resett_switch1/1, Relational Operator1/2, only_use_for_neg_speed/1, Resett_switch2/1
  Relational Operator/1 -> reset_old3/1
  Resett_switch1/1 -> Relational Operator/1, count/1, reset_old6/1
  speed_old_switch2/1 -> reset_old4/1
  Constant5/1 -> speed_old_switch2/3
  Dir/1 -> reset_old5/1
  IncsPerTurn/1 -> reset_old1/1
  Constant2/1 -> speed_old_switch2/1
  Constant3/1 -> speed_old_switch1/3
  speed_old_switch1/1 -> Add1/1
  Add1/1 -> Resett_switch2/3
  Edge/1 -> speed_old_switch1/2  "1 for one cycle if edge recognized"
  Reset/1 -> Resett_switch2/2

== system gm_Encoder_Zynq_V24/IncreEncoder_V24_Gut/omega_by_count_lines ==
  note: Count
  note: Check if count is to big in order to safe for value overflow
  note: Set new counter value
  Edge : Inport
  Reset : Inport  Port=2
  IncsPerTurn : Inport  Port=3
  Add1 : Sum  AccumDataTypeStr=int16  OutDataTypeStr=int16
  Constant1 : Constant  Value=0  OutDataTypeStr=int16  SampleTime=-1
  Constant2 : Constant  OutDataTypeStr=int16  SampleTime=-1
  Constant3 : Constant  Value=0  OutDataTypeStr=int16  SampleTime=-1
  Constant4 : Constant  Value=10  OutDataTypeStr=int16  SampleTime=-1
  Relational Operator : RelationalOperator  Operator=>  OutDataTypeStr=boolean  RndMeth=Nearest
  Reset_when_overflow : Sum  OutDataTypeStr=int16
  Resett_switch1 : Switch  Criteria=u2 ~= 0  OutDataTypeStr=int16
  Resett_switch2 : Switch  Criteria=u2 ~= 0  OutDataTypeStr=int16
  reset_old{1,3..5} (4 alike) : Delay  DelayLength=1
  reset_old_switch1 : Switch  Criteria=u2 ~= 0
  speed_old_switch1 : Switch  Criteria=u2 ~= 0
  count : Outport
  wires:
  reset_old_switch1/1 -> count/1, reset_old1/1
  Reset/1 -> Resett_switch2/2, reset_old_switch1/2  "Use new value"
  reset_old1/1 -> reset_old_switch1/3
  reset_old3/1 -> Relational Operator/1, Add1/2, reset_old_switch1/1
  Resett_switch1/1 -> reset_old3/1
  Constant4/1 -> Reset_when_overflow/1
  Constant2/1 -> reset_old4/1
  Add1/1 -> Resett_switch2/3
  IncsPerTurn/1 -> Reset_when_overflow/2
  Constant3/1 -> speed_old_switch1/3
  Constant1/1 -> Resett_switch1/1, Resett_switch2/1
  Edge/1 -> speed_old_switch1/2  "1 for one cycle if edge recognized"
  reset_old4/1 -> speed_old_switch1/1
  Resett_switch2/1 -> Resett_switch1/3
  reset_old5/1 -> Relational Operator/2
  speed_old_switch1/1 -> Add1/1
  Relational Operator/1 -> Resett_switch1/2
  Reset_when_overflow/1 -> reset_old5/1

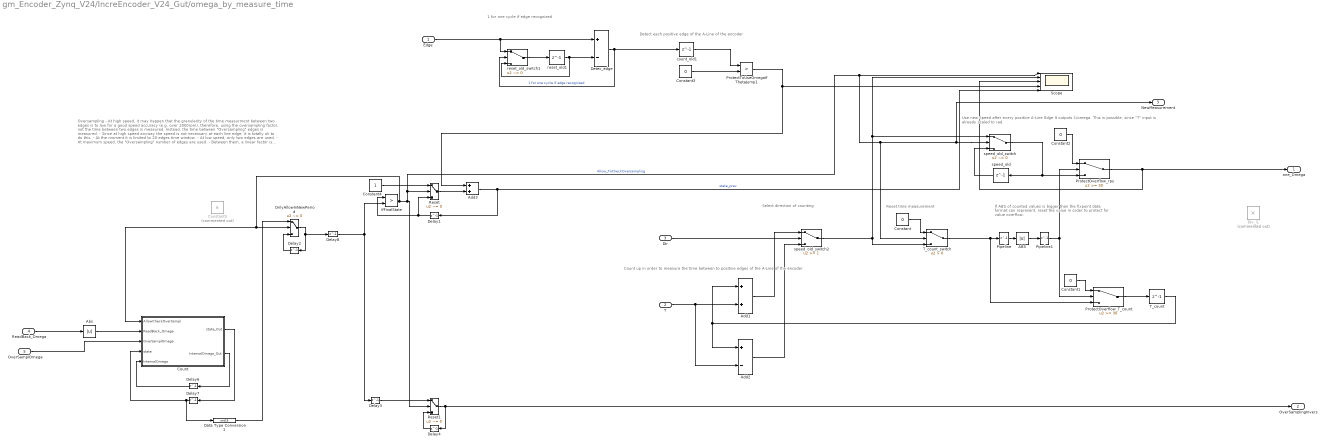
== system gm_Encoder_Zynq_V24/IncreEncoder_V24_Gut/omega_by_measure_time ==
  note: If ABS of counted values is bigger than the
      | fixpoint data format can represent, reset the
      | value in order to protect for value overflow.
  note: Select direction of counting
  note: Use new Speed after every positive A-Line Edge
      | It outputs 1/omega. This is possible, since "T" input is already scaled to rad.
  note: 1 for one cycle if edge recognized
  note: Detect each positive edge of the A-Line of the encoder
  note: Reset time measurement
  note: Count up in order to measure the time between to positive edges of the A-Line of the encoder
  note: Oversampling
      | - At high speed, it may happen that the granularity of the time measurment between
      | two edges is to low for a good speed accuracy (e.g. over 2000rpm), therefore, using
      | the oversampling factor, not the time between two edges is measured. Instead, the
      | time between "Oversampling" edges is measured.
      | - Since at high speed anyway the speed is not necessary at each line edge,
      |  it is totally ok to do this.
      | - At the moment it is limited to 20 edges time window.
      | - At low speed, only two edges are used.
      | - At maximum speed, the "Oversampling" number of edges are used.
      | - Between them, a linear factor is used.
      | - Using the OverSampling number also at low speed is not possible,
      |  since the fixpoint range must be quite high! (fixdt(1,36,30) is used at the moment)
  Edge : Inport
  T : Inport  Port=2
  Dir : Inport  Port=3
  ReadBack_Omega : Inport  Port=4
  OverSamplOmega : Inport  Port=5
  ABS : Abs
  Abs : Abs
  Add1 : Sum  OutDataTypeStr=Inherit: Same as first input
  Add2 : Sum  Inputs=+-  OutDataTypeStr=Inherit: Same as first input
  Add3 : Sum  OutDataTypeStr=Inherit: Same as accumulator
  Constant : Constant  Value=0  OutDataTypeStr=fixdt(1,36,32)  SampleTime=-1
  Constant1 : Constant  Value=0  OutDataTypeStr=fixdt(1,36,30)  SampleTime=-1
  Constant2 : Constant  Value=0  OutDataTypeStr=fixdt(1,36,32)  SampleTime=-1
  Constant3 : Constant  Value=0  OutDataTypeStr=int8  SampleTime=-1
  Constant4 : Constant  OutDataTypeStr=int8  SampleTime=T_50MHz
  Constant5 : Constant  Commented=on  Value=6  OutDataTypeStr=uint16  SampleTime=T_50MHz
  Count : MATLAB Function  TreatAsAtomicUnit=on
  Data Type Conversion1 : DataTypeConversion  OutDataTypeStr=uint16
  Delay{1..4,6,8} (6 alike) : Delay  DelayLength=1  InitialCondition=0
  Delay7 : Delay  DelayLength=1  InitialCondition=1
  Detec_edge : Sum  Inputs=+-  AccumDataTypeStr=int8  OutDataTypeStr=int8
  Div_i1 : Product  Commented=on  Inputs=**  RndMeth=Simplest  SaturateOnIntegerOverflow=on  OutDataTypeStr=Inherit: Same as first input
  IfFinalState : RelationalOperator  Operator=>  OutDataTypeStr=boolean  RndMeth=Nearest
  OnlyAllowInNewPeriod : Switch  Criteria=u2 ~= 0  Threshold=0.5  OutDataTypeStr=fixdt(0,16,0)
  Pipeline : Delay  DelayLength=1
  Pipeline1 : Delay  DelayLength=1
  ProtectOverflow_T_count : Switch  Threshold=30
  ProtectOverflow_rps : Switch  Threshold=30  OutDataTypeStr=fixdt(1,36,32)
  ProtectToUseOmegaIfThetaJump1 : RelationalOperator  Operator=>  OutDataTypeStr=fixdt(1,16)  RndMeth=Nearest
  Reset : Switch  Criteria=u2 ~= 0  Threshold=0.5  OutDataTypeStr=fixdt(1,24,11)
  Reset1 : Switch  Criteria=u2 ~= 0  Threshold=0.5  OutDataTypeStr=Inherit: Inherit via back propagation
  Scope : Scope  NumInputPorts=5
  T_count : Delay  DelayLength=1
  T_count_switch : Switch  Criteria=u2 > Threshold
  count_old1 : Delay  DelayLength=1
  reset_old1 : Delay  DelayLength=1
  reset_old_switch1 : Switch  Criteria=u2 ~= 0
  speed_old : Delay  DelayLength=1
  speed_old_switch : Switch  Criteria=u2 ~= 0  OutDataTypeStr=fixdt(1,36,32)  RndMeth=Zero
  speed_old_switch2 : Switch  Threshold=1
  one_Omega : Outport
  OverSamplingInvers : Outport  Port=2
  NewMeasurement : Outport  Port=3
  wires:
  Delay3/1 -> Reset1/1
  Abs/1 -> Count/2(ReadBack_Omega)
  Delay4/1 -> Reset1/3
  Data Type Conversion1/1 -> OnlyAllowInNewPeriod/1
  Count/1(state_Out) -> Delay7/1
  ProtectOverflow_rps/1 -> Scope/3, one_Omega/1
  Delay7/1 -> Count/4(state), Data Type Conversion1/1
  Delay6/1 -> Count/5(InternalOmega)
  Count/2(InternalOmega_Out) -> Delay6/1
  Delay2/1 -> OnlyAllowInNewPeriod/3
  OverSamplOmega/1 -> Count/3(OverSamplOmega)
  ReadBack_Omega/1 -> Abs/1
  Reset1/1 -> OverSamplingInvers/1, Delay4/1
  Delay8/1 -> Delay3/1, IfFinalState/2
  ProtectToUseOmegaIfThetaJump1/1 -> Add3/1, Scope/4
  Constant4/1 -> Reset/1
  Reset/1 -> Add3/2
  Add3/1 -> Delay1/1, Scope/5  "state_prev"
  Delay1/1 -> IfFinalState/1, Reset/3
  OnlyAllowInNewPeriod/1 -> Delay2/1, Delay8/1
  IfFinalState/1 -> OnlyAllowInNewPeriod/2, Count/1(AllowCheckOverSampl), Reset1/2, Reset/2, Scope/1, T_count_switch/2, speed_old_switch/2, NewMeasurement/1  "Allow_ToCheckOversampling"
  Pipeline1/1 -> ProtectOverflow_rps/2, ProtectOverflow_T_count/2
  Pipeline/1 -> ABS/1
  ABS/1 -> Pipeline1/1
  T_count_switch/1 -> ProtectOverflow_T_count/3, Pipeline/1
  Add2/1 -> speed_old_switch2/3
  Add1/1 -> speed_old_switch2/1
  Dir/1 -> speed_old_switch2/2
  Detec_edge/1 -> count_old1/1, reset_old_switch1/2  "1 for one cycle if edge recognized"
  reset_old1/1 -> Detec_edge/2, reset_old_switch1/3
  reset_old_switch1/1 -> reset_old1/1
  Edge/1 -> Detec_edge/1, reset_old_switch1/1
  Constant3/1 -> ProtectToUseOmegaIfThetaJump1/2
  count_old1/1 -> ProtectToUseOmegaIfThetaJump1/1
  speed_old_switch2/1 -> T_count_switch/3, speed_old_switch/1, Scope/2
  T_count/1 -> Add1/1, Add2/1
  ProtectOverflow_T_count/1 -> T_count/1
  T/1 -> Add2/2, Add1/2
  speed_old/1 -> speed_old_switch/3
  speed_old_switch/1 -> speed_old/1, ProtectOverflow_rps/3
  Constant2/1 -> ProtectOverflow_rps/1
  Constant1/1 -> ProtectOverflow_T_count/1
  Constant/1 -> T_count_switch/1

== system gm_Encoder_Zynq_V24/IncreEncoder_V24_Gut/omega_by_measure_time1 ==
  note: If ABS of counted values is bigger than the
      | fixpoint data format can represent, reset the
      | value in order to protect for value overflow.
  note: Select direction of counting
  note: Use new Speed after every positive A-Line Edge
      | It outputs 1/omega. This is possible, since "T" input is already scaled to rad.
  note: 1 for one cycle if edge recognized
  note: Detect each positive edge of the A-Line of the encoder
  note: Reset time measurement
  note: Count up in order to measure the time between to positive edges of the A-Line of the encoder
  Edge : Inport
  T : Inport  Port=2
  Dir : Inport  Port=3
  ABS : Abs
  Add1 : Sum  OutDataTypeStr=Inherit: Same as first input
  Add2 : Sum  Inputs=+-  OutDataTypeStr=Inherit: Same as first input
  Constant : Constant  Value=0  OutDataTypeStr=fixdt(1,36,30)  SampleTime=-1
  Constant1 : Constant  Value=0  OutDataTypeStr=fixdt(1,36,30)  SampleTime=-1
  Constant2 : Constant  Value=0  OutDataTypeStr=fixdt(1,36,30)  SampleTime=-1
  Constant3 : Constant  Value=0  OutDataTypeStr=int8  SampleTime=-1
  Detec_edge : Sum  Inputs=+-  AccumDataTypeStr=int8  OutDataTypeStr=int8
  Pipeline : Delay  DelayLength=1
  Pipeline1 : Delay  DelayLength=1
  ProtectOverflow_T_count : Switch  Threshold=30
  ProtectOverflow_rps : Switch  Threshold=30  OutDataTypeStr=fixdt(1,36,30)
  ProtectToUseOmegaIfThetaJump1 : RelationalOperator  Operator=>  OutDataTypeStr=boolean  RndMeth=Nearest
  Scope : Scope  NumInputPorts=3
  T_count : Delay  DelayLength=1
  T_count_switch : Switch  Criteria=u2 > Threshold
  count_old1 : Delay  DelayLength=1
  reset_old1 : Delay  DelayLength=1
  reset_old_switch1 : Switch  Criteria=u2 ~= 0
  speed_old : Delay  DelayLength=1
  speed_old_switch : Switch  Criteria=u2 ~= 0  OutDataTypeStr=fixdt(1,36,30)  RndMeth=Zero
  speed_old_switch2 : Switch  Threshold=1
  one_Omega : Outport
  NewMeasurement : Outport  Port=2
  wires:
  Pipeline1/1 -> ProtectOverflow_rps/2, ProtectOverflow_T_count/2
  Pipeline/1 -> ABS/1
  ABS/1 -> Pipeline1/1
  T_count_switch/1 -> ProtectOverflow_T_count/3, Pipeline/1
  Add2/1 -> speed_old_switch2/3
  Add1/1 -> speed_old_switch2/1
  Dir/1 -> speed_old_switch2/2
  Detec_edge/1 -> reset_old_switch1/2, count_old1/1  "1 for one cycle if edge recognized"
  reset_old1/1 -> Detec_edge/2, reset_old_switch1/3
  reset_old_switch1/1 -> reset_old1/1
  Edge/1 -> Detec_edge/1, reset_old_switch1/1
  ProtectToUseOmegaIfThetaJump1/1 -> Scope/1, T_count_switch/2, speed_old_switch/2, NewMeasurement/1
  Constant3/1 -> ProtectToUseOmegaIfThetaJump1/2
  count_old1/1 -> ProtectToUseOmegaIfThetaJump1/1
  speed_old_switch2/1 -> T_count_switch/3, speed_old_switch/1, Scope/2
  T_count/1 -> Add1/1, Add2/1
  ProtectOverflow_T_count/1 -> T_count/1
  T/1 -> Add2/2, Add1/2
  speed_old/1 -> speed_old_switch/3
  speed_old_switch/1 -> speed_old/1, ProtectOverflow_rps/3
  Constant2/1 -> ProtectOverflow_rps/1
  ProtectOverflow_rps/1 -> one_Omega/1, Scope/3
  Constant1/1 -> ProtectOverflow_T_count/1
  Constant/1 -> T_count_switch/1
